simulink model "lap2part2"  (R2021a)
settings: Solver=VariableStepAuto  StartTime=0.0  StopTime=10.0  RelTol=1e-3
settings Model: Creator=USER59  LastModifiedBy=USER59

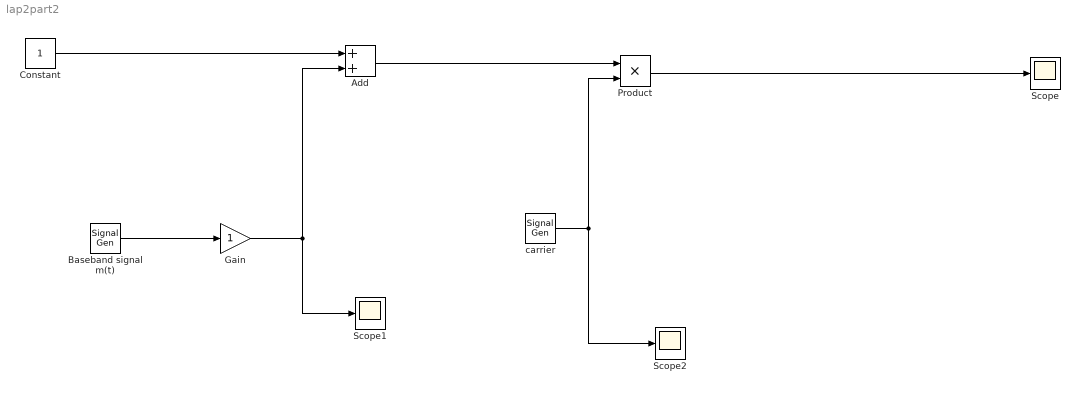
== system lap2part2 ==
  Add : Sum
  Baseband signal m(t) : SignalGenerator  Frequency=4000  Units=rad/sec
  Constant : Constant
  Gain : Gain
  Product : Product
  Scope : Scope
  Scope1 : Scope
  Scope2 : Scope
  carrier : SignalGenerator  Frequency=20000  Units=rad/sec
  wires:
  Gain/1 -> Scope1/1, Add/2
  Baseband signal m(t)/1 -> Gain/1
  Constant/1 -> Add/1
  Add/1 -> Product/1
  carrier/1 -> Scope2/1, Product/2
  Product/1 -> Scope/1
